simulink model "preview2"  (R2019a)
settings: Solver=VariableStepAuto  StartTime=0.0  StopTime=100  RelTol=1e-3
settings Model: Creator=zgz  LastModifiedBy=zgz
settings DataIOCC: ReturnWorkspaceOutputs=off

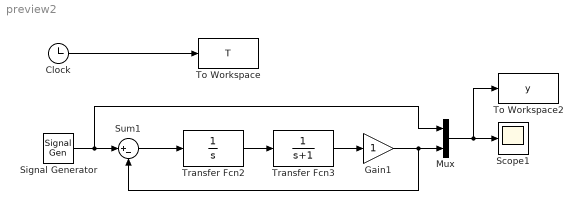
== system preview2 ==
  Clock : Clock
  Gain1 : Gain
  Mux : Mux  Inputs=2
  Scope1 : Scope
  Signal Generator : SignalGenerator  Frequency=1.292  Units=rad/sec
  Sum1 : Sum  Inputs=|+-
  To Workspace : ToWorkspace  VariableName=T  SampleTime=-1
  To Workspace2 : ToWorkspace  VariableName=y  SampleTime=-1
  Transfer Fcn2 : TransferFcn  Denominator=[1 0]
  Transfer Fcn3 : TransferFcn  Denominator=[1 1]
  wires:
  Clock/1 -> To Workspace/1
  Transfer Fcn2/1 -> Transfer Fcn3/1
  Transfer Fcn3/1 -> Gain1/1
  Signal Generator/1 -> Mux/1, Sum1/1
  Sum1/1 -> Transfer Fcn2/1
  Gain1/1 -> Mux/2, Sum1/2
  Mux/1 -> To Workspace2/1, Scope1/1
